simulink library "monroe_library"  (R2012b)
settings: Solver=ode45  StartTime=0.0  StopTime=10.0  RelTol=1e-3
values from neighbouring files (symbols this model uses):
  input_bit_width = ', num2str(input_bit_width))    [fft_direct_draw.m]
undefined symbols (not defined in the file or in its folder): gcbh, xlBlockLoadCallback
libraries: xbsIndex_r4 x1880, monroe_library x159, casper_library x13, xps_library x1
(part 24 of 43)

== system monroe_library/direct_coeff_gen/coeff_gen_stage_3_group_3 ==
  sync : Inport
  Concat : xbsIndex_r4/Concat  num_inputs=2  dbl_ovrd=off  block_type=concat
  Concat1 : xbsIndex_r4/Concat  num_inputs=2  dbl_ovrd=off  block_type=concat
  Concat2 : xbsIndex_r4/Concat  num_inputs=2  dbl_ovrd=off  block_type=concat
  Constant : xbsIndex_r4/Constant  arith_type=Boolean  const=0  n_bits=16  bin_pt=14  explicit_period=on  period=1  equ=P=C  opselect=C  inp2=PCIN>>17  opr=+  inp1=P  carry=CIN  dbl_ovrd=off  block_type=constant
  Constant1 : xbsIndex_r4/Constant  arith_type=Boolean  const=1  n_bits=16  bin_pt=14  explicit_period=off  period=1  equ=P=C  opselect=C  inp2=PCIN>>17  opr=+  inp1=P  carry=CIN  dbl_ovrd=off  block_type=constant
  Constant3 : xbsIndex_r4/Constant  arith_type=Signed (2's comp)  const=0  n_bits=18  bin_pt=17  explicit_period=on  period=1  equ=P=C  opselect=C  inp2=PCIN>>17  opr=+  inp1=P  carry=CIN  dbl_ovrd=off  block_type=constant
  Constant4 : xbsIndex_r4/Constant  arith_type=Boolean  const=0  n_bits=16  bin_pt=14  explicit_period=off  period=1  equ=P=C  opselect=C  inp2=PCIN>>17  opr=+  inp1=P  carry=CIN  dbl_ovrd=off  block_type=constant
  Constant5 : xbsIndex_r4/Constant  arith_type=Unsigned  const=2  n_bits=10  bin_pt=0  explicit_period=on  period=1  equ=P=C  opselect=C  inp2=PCIN>>17  opr=+  inp1=P  carry=CIN  dbl_ovrd=off  block_type=constant
  Counter : xbsIndex_r4/Counter  cnt_type=Free Running  cnt_to=Inf  operation=Up  start_count=0  cnt_by_val=1  arith_type=Unsigned  n_bits=10  bin_pt=0  load_pin=on  rst=off  en=off  explicit_period=on  period=1  dbl_ovrd=off  use_behavioral_HDL=off  implementation=Fabric  block_type=counter
  Delay : xbsIndex_r4/Delay  en=off  latency=0  dbl_ovrd=off  reg_retiming=off  block_type=delay
  Dual Port RAM4 : xbsIndex_r4/Dual Port RAM  depth=2048  initVector=[-0.707106781186547 -0.707648917255684 -0.708190637033195 -0.708731940200401 -0.709272826438866 -0.709813295430401 -0.710353346857062 -0.710892980401152 -0.711432195745216 -0.71197099257205 -0.712509370564692 -0.713047329406429 -0.713584868780794 -0.714121988371565 -0.714658687862769 -0.71519496693868 -0.715730825283819 -0.716266262582953 -0.716801278521099 -0.717335872783522 -0.717870045055732 -0.71840379502349 -0.718937122372804 -0.719470026789933 -0.720002507961382 -0.720534565573905 -0.721066199314508 -0.721597408870444 -0.722128193929215 -0.722658554178576 -0.723188489306527 -0.723717999001323 -0.724247082951467 -0.724775740845711 -0.725303972373061 -0.72583177722277 -0.726359155084346 -0.726886105647545 -0.727412628602376 -0.727938723639099 -0.728464390448225 -0.728989628720519 -0.729514438146997 -0.730038818418926 -0.730562769227828 -0.731086290265474 -0.731609381223893 -0.732132041795361 -0.732654271672413 -0.733176070547833 -0.73369743811466 -0.734218374066188 -0.734738878095963 -0.735258949897787 -0.735778589165713 -0.736297795594053 -0.73681656887737 -0.737334908710483 -0.737852814788466 -0.738370286806649 -0.738887324460615 -0.739403927446206 -0.739920095459516 -0.740435828196898 -0.740951125354959 -0.741465986630563 -0.741980411720831 -0.742494400323139 -0.743007952135122 -0.743521066854669 -0.744033744179929 -0.744545983809307 -0.745057785441466 -0.745569148775325 -0.746080073510064 -0.746590559345117 -0.74710060598018 -0.747610213115205 -0.748119380450404 -0.748628107686245 -0.749136394523459 -0.749644240663033 -0.750151645806215 -0.750658609654511 -0.751165131909686 -0.751671212273768 -0.752176850449043 -0.752682046138055 -0.753186799043613 -0.753691108868781 -0.754194975316889 -0.754698398091525 -0.755201376896537 -0.755703911436036 -0.756206001414395 -0.756707646536246 -0.757208846506485 -0.757709601030268 -0.758209909813015 -0.758709772560407 -0.759209188978388 -0.759708158773163 -0.760206681651202 -0.760704757319237 -0.761202385484262 -0.761699565853535 -0.762196298134579 -0.762692582035178 -0.763188417263381 -0.763683803527502 -0.764178740536117 -0.764673227998067 -0.765167265622459 -0.765660853118662 -0.766153990196313 -0.76664667656531 -0.76713891193582 -0.767630696018273 -0.768122028523365 -0.768612909162058 -0.76910333764558 -0.769593313685423 -0.770082836993348 -0.770571907281381 -0.771060524261814 -0.771548687647206 -0.772036397150384 -0.772523652484441 -0.773010453362737 -0.773496799498899 -0.773982690606823 -0.774468126400671 -0.774953106594874 -0.775437630904131 -0.775921699043408 -0.77640531072794 -0.776888465673232 -0.777371163595056 -0.777853404209453 -0.778335187232733 -0.778816512381476 -0.77929737937253 -0.779777787923014 -0.780257737750317 -0.780737228572094 -0.781216260106276 -0.781694832071059 -0.782172944184913 -0.782650596166576 -0.783127787735057 -0.783604518609638 -0.78408078850987 -0.784556597155575 -0.785031944266848 -0.785506829564054 -0.78598125276783 -0.786455213599086 -0.786928711779002 -0.787401747029031 -0.7878743190709 -0.788346427626606 -0.78881807241842 -0.789289253168886 -0.789759969600819 -0.79023022143731 -0.790700008401722 -0.79116933021769 -0.791638186609126 -0.792106577300212 -0.792574502015408 -0.793041960479444 -0.793508952417327 -0.793975477554337 -0.794441535616031 -0.794907126328237 -0.795372249417061 -0.795836904608884 -0.796301091630359 -0.796764810208419 -0.797228060070269 -0.797690840943391 -0.798153152555544 -0.798614994634761 -0.799076366909352 -0.799537269107905 -0.799997700959282 -0.800457662192623 -0.800917152537344 -0.80137617172314 -0.801834719479981 -0.802292795538116 -0.802750399628069 -0.803207531480645 -0.803664190826924 -0.804120377398266 -0.804576090926307 -0.805031331142964 -0.805486097780429 -0.805940390571176 -0.806394209247956 -0.806847553543799 -0.807300423192014 -0.80775281792619 -0.808204737480195 -0.808656181588175 -0.809107149984558 -0.809557642404051 -0.810007658581641 -0.810457198252595 -0.81090626115246 -0.811354847017064 ...(+33801 chars)]  distributed_mem=Block RAM  init_a=0  init_b=0  rst_a=off  rst_b=off  en_a=off  en_b=off  latency=2  write_mode_A=No Read On Write  write_mode_B=No Read On Write  dbl_ovrd=off  optimize=Area  use_rpm=on  block_type=dpram
  Reinterpret : xbsIndex_r4/Reinterpret  force_arith_type=on  arith_type=Unsigned  force_bin_pt=on  bin_pt=0  block_type=reinterpret
      settings: infoedit="Changes signal type without altering the binary representation.   You can changed the signal between signed and unsigned, and relocate the binary point.<br><br>Hardware notes: In hardware this block costs nothing.<br><br>Example:  Suppose the input is 6 bits wide, signed, with 2 fractional bits, and the output is forced to unsigned with 0 fractional bits.  Then an input of -2.0 (1110.00 in binary 2's complement) becomes an output of 56 (111000 in binary)."
  Reinterpret1 : xbsIndex_r4/Reinterpret  force_arith_type=on  arith_type=Unsigned  force_bin_pt=on  bin_pt=0  block_type=reinterpret
      settings: infoedit="Changes signal type without altering the binary representation.   You can changed the signal between signed and unsigned, and relocate the binary point.<br><br>Hardware notes: In hardware this block costs nothing.<br><br>Example:  Suppose the input is 6 bits wide, signed, with 2 fractional bits, and the output is forced to unsigned with 0 fractional bits.  Then an input of -2.0 (1110.00 in binary 2's complement) becomes an output of 56 (111000 in binary)."
  count_slice : xbsIndex_r4/Slice  nbits=10  boolean_output=off  mode=Upper Bit Location + Width  bit1=0  base1=MSB of Input  bit0=0  base0=MSB of Input  dbl_ovrd=off  block_type=slice
  coeff : Outport
  wires:
  count_slice/1 -> Concat1/2, Concat/2  "xlsub2_Counter_out1"
  Constant3/1 -> Dual Port RAM4/5, Dual Port RAM4/2  "xlsub2_Constant3_out1"
  Constant/1 -> Dual Port RAM4/6, Dual Port RAM4/3  "xlsub2_Constant_out1"
  Reinterpret1/1 -> Concat2/2  "xlsub2_Reinterpret1_out1"
  Dual Port RAM4/2 -> Reinterpret1/1  "xlsub2_Dual_Port_RAM4_out2"
  Reinterpret/1 -> Concat2/1  "xlsub2_Reinterpret_out1"
  Dual Port RAM4/1 -> Reinterpret/1  "xlsub2_Dual_Port_RAM4_out1"
  Concat1/1 -> Dual Port RAM4/4  "xlsub2_Concat1_out1"
  Concat/1 -> Dual Port RAM4/1  "xlsub2_Concat_out1"
  Delay/1 -> coeff/1
  Concat2/1 -> Delay/1  "xlsub2_Concat2_out1"
  Counter/1 -> count_slice/1
  Constant5/1 -> Counter/2  "xlsub2_Constant5_out1"
  sync/1 -> Counter/1
  Constant4/1 -> Concat1/1  "xlsub2_Constant4_out1"
  Constant1/1 -> Concat/1  "xlsub2_Constant1_out1"
